simulink library "odm_wheel"  (R2020b)
settings: Solver=VariableStepAuto  StartTime=0.0  StopTime=10.0  RelTol=1e-3
settings Model: Creator=tfpeng  LastModifiedBy=tfpeng

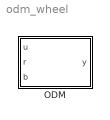
== system odm_wheel ==
  ODM : MATLAB Function  TreatAsAtomicUnit=on

== matlab function odm_wheel/ODM ==
  data: u input; y output; r input; b input
function y = odometry_wheel(u,r,b)
persistent state_current;
if isempty(state_current)
   state_current=zeros(3,1);%(x,y,theta)
end
v=(u(1)+u(2))*r/2;
w=(u(2)-u(1))*r/2/b;
dt=0.01;
d=v*dt;
dx=d*cos(state_current(3)+w*dt/2);
dy=d*sin(state_current(3)+w*dt/2);
state_current(3)=state_current(3)+w*dt;
state_current(1)=state_current(1)+dx;
state_current(2)=state_current(2)+dy;
y = state_current;
